simulink model "L_10_12_sim24bMPC"  (R2024b)
settings: Solver=ode45  StartTime=0.0  StopTime=t_sim  MaxStep=0.0001*Ts  MinStep=0.00001*Ts  RelTol=1e-3  EnableMultiTasking=on
values from neighbouring files (symbols this model uses):
  C = [1 0]    [Es1_l7.m]    (also in Lab_Practice_7_1.m; Lab_Practice_7_1.mat; MPC_example_10_12.m = [600 0]; MPC_ratevariation.m = [600 0])
  md = MPCInit(Ad,Bd,Cy,Cz,Dz,Cc,Dc,Hp,Hw,z_blk,Hu,u_blk,du_max,du_min,u_max,u_min,z_max,z_min,Q,R,[],[],h,cmode,'qp_as')    [Es1_l7.m]    (also in Lab_Practice_7_1.m = MPCInit(Ad,Bd,Cy,Cz,Dz,Cc,Dc,Hp,Hw, z_blk, Hc, u_blk, du_max; Lab_Practice_7_1.mat = ; MPC_example_10_12.m; MPC_ratevariation.m)
  rho = 1    [Es1_l7.m]    (also in MPC_example_10_12.m; MPC_zeroregulation.m)
  Ts = 0.05    [Es1_l7.m]    (also in Lab_Practice_7_1.m; Lab_Practice_7_1.mat; MPC_example_10_12.m = 0.001; MPC_ratevariation.m = 0.001)
  x0 = [1; 0]    [Es1_l7.m]    (also in Lab_Practice_7_1.m = [1;0]; Lab_Practice_7_1.mat = [1 0]; MPC_example_10_12.m = [0;0]; MPC_ratevariation.m = [-0.25;0])
libraries: cstblocks x1
settings Model: Creator=jakesson  LastModifiedBy=filoz
settings SolverCC: InitialStep=0.00001*Ts  AlgebraicLoopSolver=TrustRegion
settings DataIOCC: LimitDataPoints=on  SaveFormat=Array  SignalLoggingSaveFormat=ModelDataLogs  ReturnWorkspaceOutputs=off  SignalLoggingName=sigsOut
settings OptimizationCC: BooleanDataType=off  InitFltsAndDblsToZero=on  LifeSpan=inf
settings DebuggingCC: SaveWithParameterizedLinksMsg=none  UnderspecifiedInitializationDetection=Classic  MergeDetectMultiDrivingBlocksExec=none  SignalResolutionControl=TryResolveAllWithWarning  MultiTaskDSMMsg=warning  MultiTaskCondExecSysMsg=none  FcnCallInpInsideContextMsg=warning  UnconnectedInputMsg=warning  UnconnectedOutputMsg=warning  UnconnectedLineMsg=warning  AllowSymbolicDim=off  SFUnexpectedBacktrackingDiag=warning  SFNoUnconditionalDefaultTransitionDiag=warning  SFExecutionAtInitializationDiag=none  ArithmeticOperatorsInVariantConditions=warning
settings HardwareCC: ProdBitPerPointer=32  ProdBitPerSizeT=32  ProdBitPerPtrDiffT=32  ProdLargestAtomicFloat=None  ProdIntDivRoundTo=Undefined  ProdEndianess=Unspecified  ProdWordSize=32  ProdHWDeviceType=32-bit Generic  TargetUnknown=on
settings ModelReferenceCC: EnableRefExpFcnMdlSchedulingChecks=on  PropagateSignalLabelsOutOfModel=off
settings SFSimCC: SimUseLocalCustomCode=off  CustomCodeUndefinedFunction=UseInterfaceOnly
settings RTWCC: RTWUseLocalCustomCode=off  GPUComputeCapability=3.5
settings CodeAppCC: StateflowObjectComments=on
settings GRTTargetCC: TargetFcnLib=ansi_tfl_tmw.mat  TargetLangStandard=C89/C90 (ANSI)  CombineOutputUpdateFcns=off  GRTInterface=on
settings ConfigComp: CovMetricSettings=dw  CovSaveCumulativeToWorkspaceVar=on  CovSaveSingleToWorkspaceVar=on  CovExternalEMLEnable=off

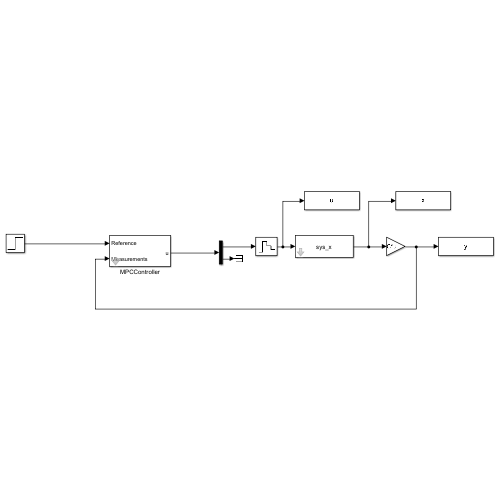
[thumbnail: Simulink's stored preview of the top-level diagram]
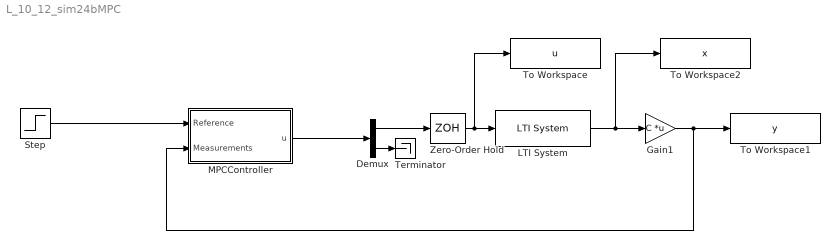
== system L_10_12_sim24bMPC ==
  Demux : Demux  Outputs=2
  Gain1 : Gain  Gain=C  Multiplication=Matrix(K*u)
  LTI System : cstblocks/LTI System  sys=sys_x  IC=[x0]  PadeOrder=0
  MPCController : Subsystem  mask{md=md}
      mask prompts: md "MPCData"
  Step : Step  Time=0  After=rho  SampleTime=Ts
  Terminator : Terminator
  To Workspace : ToWorkspace  VariableName=u  SaveFormat=Timeseries  SampleTime=Ts
  To Workspace1 : ToWorkspace  VariableName=y  SaveFormat=Timeseries  SampleTime=Ts
  To Workspace2 : ToWorkspace  VariableName=x  SaveFormat=Timeseries  SampleTime=Ts
  Zero-Order Hold : ZeroOrderHold  SampleTime=Ts
  wires:
  Step/1 -> MPCController/1(Reference)
  MPCController/1(u) -> Demux/1
  Demux/1 -> Zero-Order Hold/1
  Demux/2 -> Terminator/1
  Zero-Order Hold/1 -> To Workspace/1, LTI System/1
  LTI System/1 -> To Workspace2/1, Gain1/1
  Gain1/1 -> MPCController/2(Measurements), To Workspace1/1

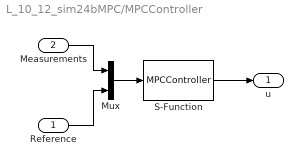
== system L_10_12_sim24bMPC/MPCController ==
  Reference : Inport
  Measurements : Inport  Port=2
  Mux : Mux  Inputs=2
  S-Function : S-Function  FunctionName=MPCController  Parameters=md  SFunctionDeploymentMode=off  EnableBusSupport=off
  u : Outport
  wires:
  Mux/1 -> S-Function/1
  Measurements/1 -> Mux/1
  Reference/1 -> Mux/2
  S-Function/1 -> u/1
